simulink model "motorEncoder"  (R2017a)
settings: Solver=VariableStepAuto  StartTime=0.0  StopTime=60  RelTol=1e-3
libraries: arduino_io_lib x4
settings Model: Creator=enes_  LastModifiedBy=enes_

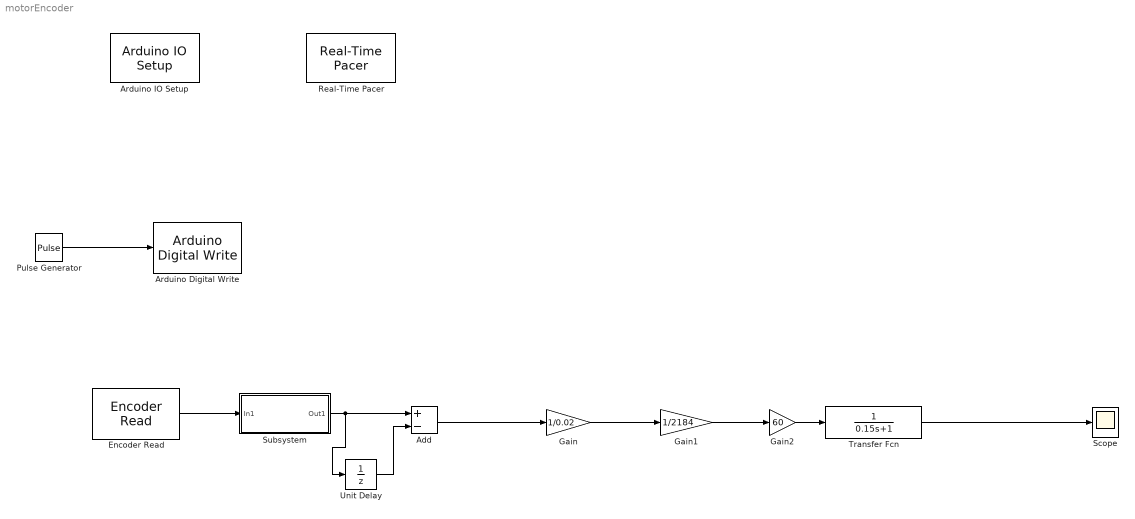
== system motorEncoder ==
  Add : Sum  Inputs=+-
  Arduino Digital Write : arduino_io_lib/Arduino Digital Write  arduinoVar=Temporary arduino variable: Arduino1  arduinoPin=5  T=-1
  Arduino IO Setup : arduino_io_lib/Arduino IO Setup  Priority=3  arduinoVar=Temporary arduino variable: Arduino1  workspaceVarName=a  comPort=COM4
  Encoder Read : arduino_io_lib/Encoder Read  arduinoVar=Temporary arduino variable: Arduino1  encNum=1  pinA=2  pinB=3  DbDl=0  T=0.02
  Gain : Gain  Gain=1/0.02
  Gain1 : Gain  Gain=1/2184
  Gain2 : Gain  Gain=60
  Pulse Generator : DiscretePulseGenerator  Period=28/0.02  PulseWidth=28/0.02  PhaseDelay=2/0.02  SampleTime=0.02
  Real-Time Pacer : arduino_io_lib/Real-Time Pacer  simTimePerRealTime=1
  Scope : Scope
  Subsystem : Subsystem
  Transfer Fcn : TransferFcn  Denominator=[0.15 1]
  Unit Delay : UnitDelay  SampleTime=-1
  wires:
  Pulse Generator/1 -> Arduino Digital Write/1
  Encoder Read/1 -> Subsystem/1(In1)
  Subsystem/1(Out1) -> Unit Delay/1, Add/1
  Unit Delay/1 -> Add/2
  Add/1 -> Gain/1
  Gain/1 -> Gain1/1
  Gain1/1 -> Gain2/1
  Gain2/1 -> Transfer Fcn/1
  Transfer Fcn/1 -> Scope/1

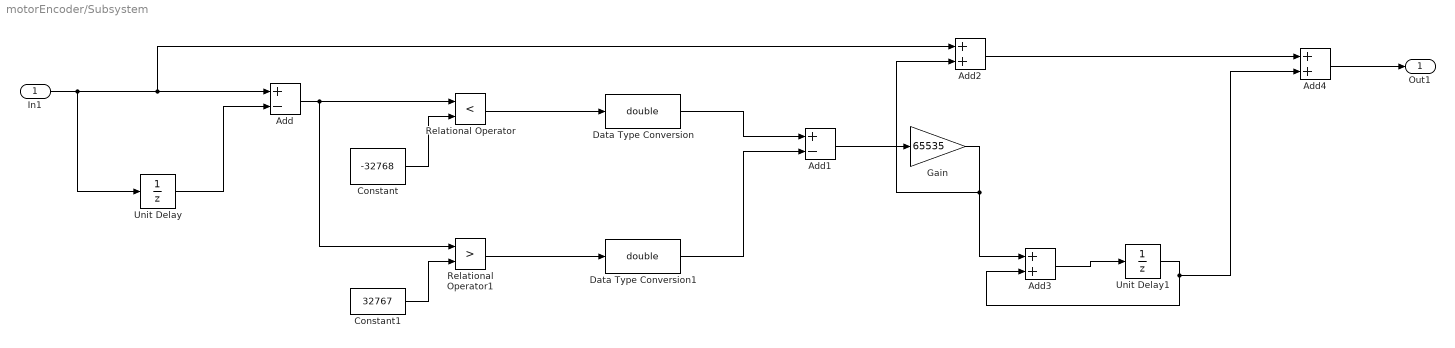
== system motorEncoder/Subsystem ==
  In1 : Inport
  Add : Sum  Inputs=+-
  Add1 : Sum  Inputs=+-
  Add2 : Sum
  Add3 : Sum
  Add4 : Sum
  Constant : Constant  Value=-32768
  Constant1 : Constant  Value=32767
  Data Type Conversion : DataTypeConversion  OutDataTypeStr=double
  Data Type Conversion1 : DataTypeConversion  OutDataTypeStr=double
  Gain : Gain  Gain=65535
  Relational Operator : RelationalOperator  Operator=<  OutDataTypeStr=boolean  RndMeth=Simplest
  Relational Operator1 : RelationalOperator  Operator=>  OutDataTypeStr=boolean  RndMeth=Simplest
  Unit Delay : UnitDelay  SampleTime=-1
  Unit Delay1 : UnitDelay  SampleTime=-1
  Out1 : Outport
  wires:
  In1/1 -> Add2/1, Add/1, Unit Delay/1
  Unit Delay/1 -> Add/2
  Constant/1 -> Relational Operator/2
  Add/1 -> Relational Operator1/1, Relational Operator/1
  Constant1/1 -> Relational Operator1/2
  Relational Operator1/1 -> Data Type Conversion1/1
  Relational Operator/1 -> Data Type Conversion/1
  Data Type Conversion/1 -> Add1/1
  Data Type Conversion1/1 -> Add1/2
  Add1/1 -> Gain/1
  Add2/1 -> Add4/1
  Gain/1 -> Add3/1, Add2/2
  Add4/1 -> Out1/1
  Add3/1 -> Unit Delay1/1
  Unit Delay1/1 -> Add4/2, Add3/2
